simulink model "visualize_imu"  (Simulink 8.3)
settings: Solver=FixedStepDiscrete  StartTime=0.0  StopTime=inf  FixedStep=0.01  RelTol=1e-3
libraries: WBToolboxLibrary x2
settings Model: Creator=The MathWorks, Inc.  LastModifiedBy=gabri
settings DataIOCC: SaveFormat=Dataset  SignalLoggingSaveFormat=Dataset
settings DebuggingCC: UnderspecifiedInitializationDetection=Simplified  MergeDetectMultiDrivingBlocksExec=error  SolverPrmCheckMsg=none  FrameProcessingCompatibilityMsg=error  StateNameClashWarn=none
settings HardwareCC: ProdBitPerPointer=64  ProdLargestAtomicFloat=Float  ProdIntDivRoundTo=Zero  ProdEndianess=LittleEndian  ProdWordSize=64  ProdHWDeviceType=Intel->x86-64 (Windows64)
settings GRTTargetCC: GeneratePreprocessorConditionals=Use local settings  CombineOutputUpdateFcns=on  GRTInterface=off
settings ConfigComp: CovMetricSettings=dw  CovHtmlReporting=on  CovSaveCumulativeToWorkspaceVar=on  CovSaveSingleToWorkspaceVar=on  CovExternalEMLEnable=off

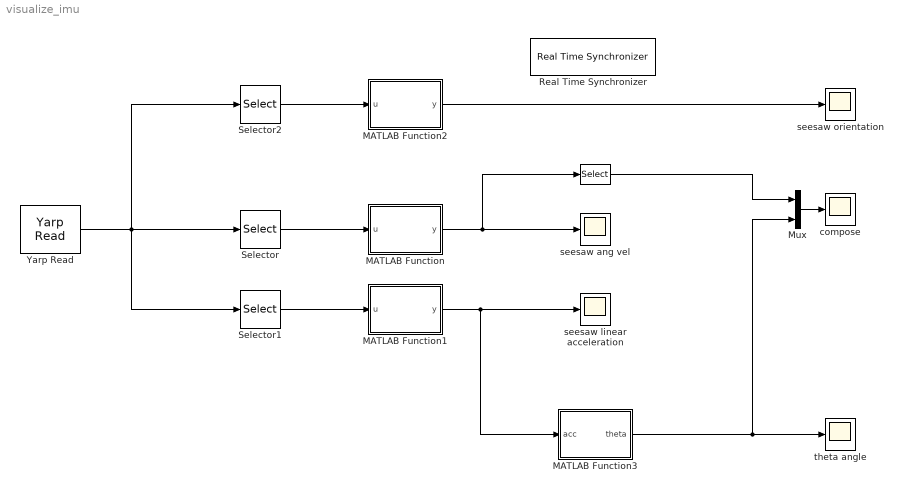
== system visualize_imu ==
  " " : Selector  InputPortWidth=3  Indices=[1]
  MATLAB Function : MATLAB Function  TreatAsAtomicUnit=on
  MATLAB Function1 : MATLAB Function  TreatAsAtomicUnit=on
  MATLAB Function2 : MATLAB Function  TreatAsAtomicUnit=on
  MATLAB Function3 : MATLAB Function  TreatAsAtomicUnit=on
  Mux : Mux  Inputs=2
  Real Time Synchronizer : WBToolboxLibrary/Utilities/Real Time Synchronizer  period=0.01
  Selector : Selector  InputPortWidth=9  Indices=[7 8 9]
  Selector1 : Selector  InputPortWidth=9  Indices=[4 5 6]
  Selector2 : Selector  InputPortWidth=9  Indices=[1 2 3]
  Yarp Read : WBToolboxLibrary/Utilities/Yarp Read  portName='/seesaw'  signalSize=9  blocking=off  timestamp=off  autoconnect=on  errorOnConnection=on
  compose : Scope
  seesaw ang vel : Scope
  seesaw linear acceleration : Scope
  seesaw orientation : Scope
  theta angle : Scope
  wires:
  Yarp Read/1 -> Selector2/1, Selector/1, Selector1/1
  Selector/1 -> MATLAB Function/1(u)
  MATLAB Function/1(y) -> " "/1, seesaw ang vel/1
  Selector1/1 -> MATLAB Function1/1(u)
  MATLAB Function1/1(y) -> seesaw linear acceleration/1, MATLAB Function3/1(acc)
  Selector2/1 -> MATLAB Function2/1(u)
  MATLAB Function2/1(y) -> seesaw orientation/1
  Mux/1 -> compose/1
  MATLAB Function3/1(theta) -> theta angle/1, Mux/2
  " "/1 -> Mux/1

== matlab function MATLAB Function1 ==
  data: u input double; y output double
function y = rotate(u)

y = rotx(pi)*rotz(-44/180*pi)*u;

end

== matlab function MATLAB Function ==
  data: u input double; y output double
function y = rotate(u)

y = rotx(pi)*rotz(-44/180*pi)*u;

end

== matlab function MATLAB Function2 ==
  data: u input double; y output double
function y = rotate(u)

y = rotx(pi)*rotz(-44/180*pi)*u;

end

== matlab function MATLAB Function3 ==
  data: acc input double; theta output double
function theta = arctangent(acc)

theta = atan2(acc(2),acc(3))*180/pi;

end
